simulink model "iPendulumHinf"  (R2019a)
settings: Solver=ode23s  StartTime=0.0  StopTime=10  MaxStep=0.12  RelTol=1e-3
undefined symbols (not defined in the file): K_inf, normalize_u, normalize_y, r_dphi, u_dist
libraries: iPendulumLibrary x2
settings Model: Creator=Chris  LastModifiedBy=Marlin Siebert
settings DataIOCC: ReturnWorkspaceOutputs=off
settings DebuggingCC: ArithmeticOperatorsInVariantConditions=warning
settings SFSimCC: SimUseLocalCustomCode=off
settings RTWCC: RTWUseLocalCustomCode=off
settings CodeAppCC: StateflowObjectComments=on

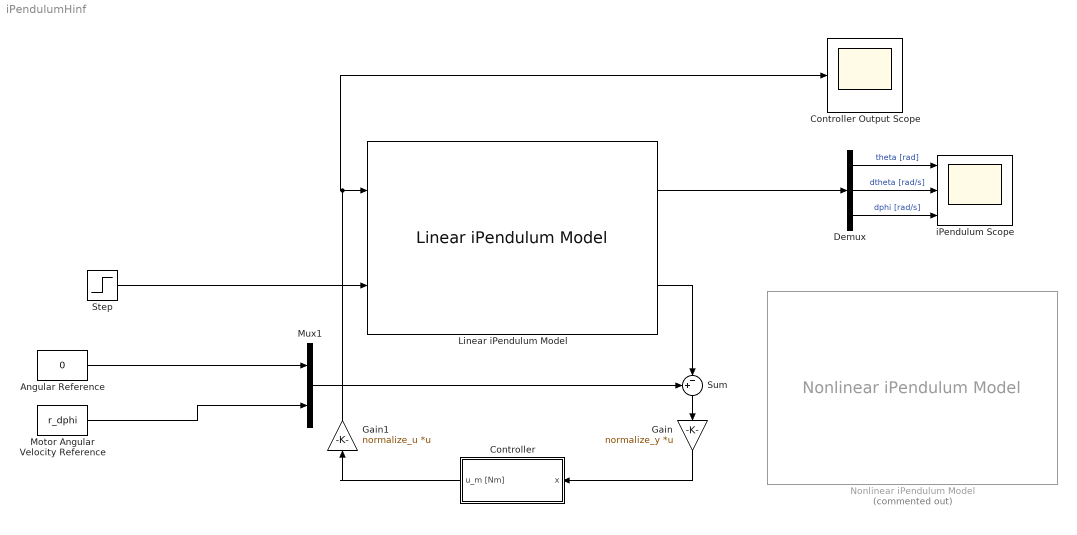
== system iPendulumHinf ==
  Angular Reference : Constant  Value=0
  Controller : Subsystem
  Controller Output Scope : Scope
  Demux : Demux  Outputs=3
  Gain : Gain  Gain=normalize_y  Multiplication=Matrix(K*u) (u vector)
  Gain1 : Gain  Gain=normalize_u  Multiplication=Matrix(K*u) (u vector)
  Linear iPendulum Model : iPendulumLibrary/Linear iPendulum Model  SystemSampleTime=-1
  Motor Angular Velocity Reference : Constant  Value=r_dphi
  Mux1 : Mux  Inputs=2
  Nonlinear iPendulum Model : iPendulumLibrary/Nonlinear iPendulum Model  Commented=on  SystemSampleTime=-1
  Step : Step  Time=5  After=u_dist  SampleTime=0
  Sum : Sum  Inputs=+-|
  iPendulum Scope : Scope  NumInputPorts=3
  wires:
  Angular Reference/1 -> Mux1/1
  Linear iPendulum Model/1 -> Demux/1
  Demux/2 -> iPendulum Scope/2  "dtheta [rad/s]"
  Demux/1 -> iPendulum Scope/1  "theta [rad]"
  Demux/3 -> iPendulum Scope/3  "dphi [rad/s]"
  Mux1/1 -> Sum/1
  Controller/1(u_m [Nm]) -> Gain1/1
  Sum/1 -> Gain/1
  Step/1 -> Linear iPendulum Model/2
  Gain/1 -> Controller/1(x)
  Gain1/1 -> Linear iPendulum Model/1, Controller Output Scope/1
  Linear iPendulum Model/2 -> Sum/2
  Motor Angular Velocity Reference/1 -> Mux1/2

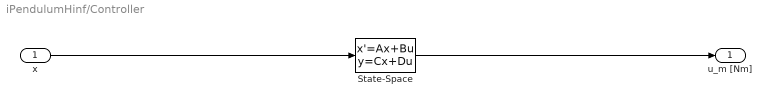
== system iPendulumHinf/Controller ==
  x : Inport
  State-Space : StateSpace  A=K_inf.a  B=K_inf.b  C=K_inf.c  D=K_inf.d  InitialCondition=0
  u_m [Nm] : Outport
  wires:
  x/1 -> State-Space/1
  State-Space/1 -> u_m [Nm]/1
